simulink model "rampinputnuke"  (R2014a)
settings: Solver=ode45  StartTime=0.0  StopTime=10.0  RelTol=1e-3
settings Model: Creator=wangwenchen  LastModifiedBy=wangwenchen

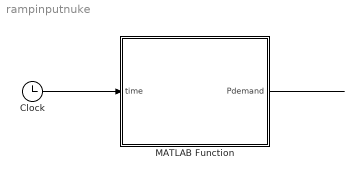
== system rampinputnuke ==
  Clock : Clock
  MATLAB Function : MATLAB Function  TreatAsAtomicUnit=on
  wires:
  Clock/1 -> MATLAB Function/1(time)
  MATLAB Function/1(Pdemand) -> ?

== matlab function rampinputnuke/MATLAB Function ==
  data: time input; Pdemand output
function Pdemand = rampnuke(time)
%#codegen

Pdemand = 37.8 + 4.2/120 * time;

return
